simulink model "dynamics"  (R2016a)
settings: Solver=VariableStepAuto  StartTime=0.0  StopTime=10.0  RelTol=1e-3
settings Model: Creator=hugoa  LastModifiedBy=ALEX

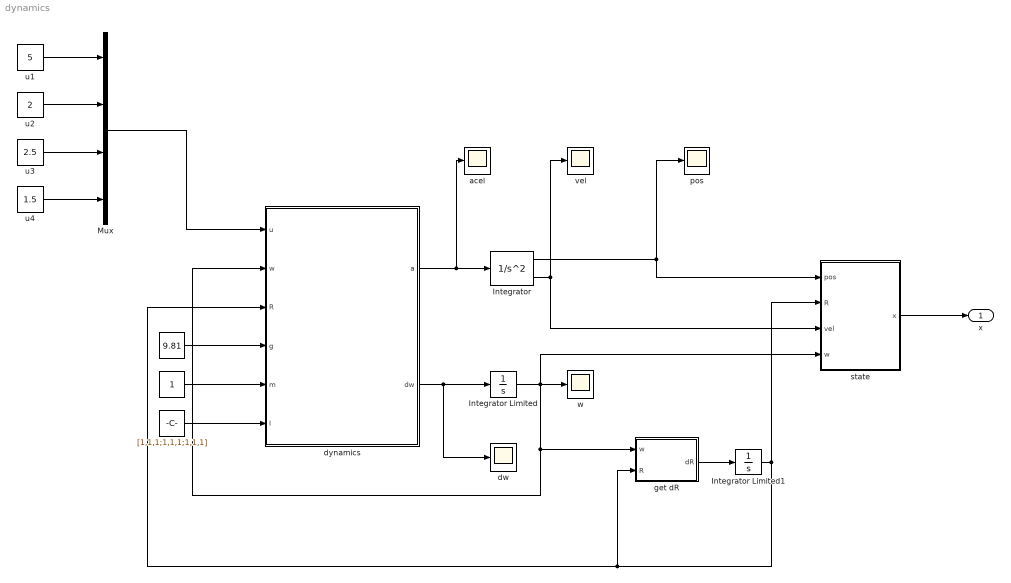
== system dynamics ==
  " " : Constant
  " " : Constant  Value=[1,1,1;1,1,1;1,1,1]
  " " : Constant  Value=9.81
  " u1 " : Constant  Value=5
  " u2" : Constant  Value=2
  " u3" : Constant  Value=2.5
  " u4" : Constant  Value=1.5
  Integrator : SecondOrderIntegrator  LimitX=on  UpperLimitX=1  LowerLimitX=0  LimitDXDT=on
  Integrator Limited : Integrator  LimitOutput=on  UpperSaturationLimit=1  LowerSaturationLimit=0
  Integrator Limited1 : Integrator  LimitOutput=on  UpperSaturationLimit=1  LowerSaturationLimit=0
  Mux : Mux
  acel : Scope
  dw : Scope
  dynamics : MATLAB Function  TreatAsAtomicUnit=on
  get dR : MATLAB Function  TreatAsAtomicUnit=on
  pos : Scope
  state : MATLAB Function  TreatAsAtomicUnit=on
  vel : Scope
  w : Scope
  x : Outport
  wires:
  dynamics/1(a) -> acel/1, Integrator/1
  dynamics/2(dw) -> dw/1, Integrator Limited/1
  " "/1 -> dynamics/4(g)
  " "/1 -> dynamics/6(I)
  " "/1 -> dynamics/5(m)
  Integrator Limited/1 -> state/4(w), dynamics/2(w), get dR/1(w), w/1
  Integrator/1 -> state/1(pos), pos/1
  Integrator/2 -> vel/1, state/3(vel)
  get dR/1(dR) -> Integrator Limited1/1
  Integrator Limited1/1 -> state/2(R), get dR/2(R), dynamics/3(R)
  state/1(x) -> x/1
  Mux/1 -> dynamics/1(u)
  " u1 "/1 -> Mux/1
  " u2"/1 -> Mux/2
  " u3"/1 -> Mux/3
  " u4"/1 -> Mux/4

== matlab function dynamics/get dR ==
  data: w input; dR output; R input
function dR = fcn(w, R)
%#codegen
skew_w = zeros(3);
skew_w = skew_w + [0, -w(1), w(2); w(2), 0, -w(1); -w(3), w(1), 0];

dR = R*skew_w;

== matlab function dynamics/dynamics ==
  data: u input; a output; w input; R input; g input; m input; I input; dw output
function [a,dw] = fcn(u,w, R, g, m, I)
%#codegen
zw = transpose([0 0 1]);
skew_w = zeros(3);
skew_w = skew_w + [0 -w(1) w(2); w(2) 0 -w(1); -w(3) w(1) 0];
zB = R*zw;
a = -g*zw+(u(1)/m)*zB;
dw = zeros(3);

dw = dw + inv(I)*(-skew_w*I*w*+u);

== matlab function dynamics/state ==
  data: pos input; R input; vel input; w input; x output
function x = fcn(pos, R, vel, w)
%#codegen

x = [pos, vel, w, R];
